simulink model "SSi_tracking_test_2024"  (R2024b)
settings: Solver=ode1  StartTime=0.0  StopTime=10  FixedStep=0.002  RelTol=1e-3  EnableMultiTasking=on
PostLoadFcn:
  | qc_set_target_type(getConfigSet(bdroot, 'QUARC Default Target Configuration'));
undefined symbols (not defined in the file): Aobs_d, Bobs_d, Cobs_d, Dobs_d, HIL, init_cond4, K5d, ud_neg, ud_pos, V_sat
libraries: quarc_library x4, simulink_extras x1
settings Model: SimulationMode=external  ExtModeTrigDuration=5000  Creator=pmartin  LastModifiedBy=Student
settings SolverCC: AlgebraicLoopSolver=TrustRegion  PositivePriorityOrder=on
settings DataIOCC: LimitDataPoints=on  SaveFormat=Array  SignalLoggingSaveFormat=ModelDataLogs  ReturnWorkspaceOutputs=off
settings OptimizationCC: ExpressionDepthLimit=2147483647  InitFltsAndDblsToZero=on
settings DebuggingCC: SaveWithParameterizedLinksMsg=none  UnderspecifiedInitializationDetection=Classic  MergeDetectMultiDrivingBlocksExec=none  SolverPrmCheckMsg=warning  MultiTaskDSMMsg=warning  MultiTaskCondExecSysMsg=none  FcnCallInpInsideContextMsg=warning  UnconnectedInputMsg=warning  UnconnectedOutputMsg=warning  UnconnectedLineMsg=warning  StateNameClashWarn=warning  SFUnexpectedBacktrackingDiag=warning  SFNoUnconditionalDefaultTransitionDiag=warning  SFExecutionAtInitializationDiag=none  ArithmeticOperatorsInVariantConditions=warning
settings ModelReferenceCC: PropagateSignalLabelsOutOfModel=off
settings SFSimCC: SimUseLocalCustomCode=off  CustomCodeUndefinedFunction=UseInterfaceOnly
settings RTWCC: Description=QUARC Win64 Target Using Toolchain  SystemTargetFile=quarc_win64.tlc  TemplateMakefile=quarc_default_tmf  RTWUseLocalCustomCode=off  Toolchain=QUARC win64 | nmake (64-bit Windows)  BuildConfiguration=Faster Runs  GPUComputeCapability=3.5
settings CodeAppCC: StateflowObjectComments=on
settings STFCustomTargetCC: ModelReferenceCompliant=off  CombineOutputUpdateFcns=on  MatFileLogging=on  UseToolchainInfoCompliant=on  SystemTargetFile=quarc_win64.tlc
settings GRTTargetCC: TargetLangStandard=C89/C90 (ANSI)  ModelReferenceCompliant=off  ParMdlRefBuildCompliant=off  CompOptLevelCompliant=off  ConcurrentExecutionCompliant=off  CPPClassGenCompliant=off  ExtMode=on  ExtModeMexFile=quarc_comm  ExtModeMexArgs='-w -uri %u'
settings ConfigComp: CovMetricSettings=dw  CovSaveCumulativeToWorkspaceVar=on  CovSaveSingleToWorkspaceVar=on  CovExternalEMLEnable=off

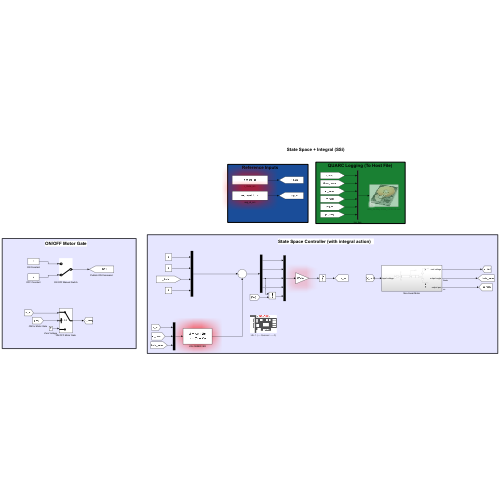
[thumbnail: Simulink's stored preview of the top-level diagram]
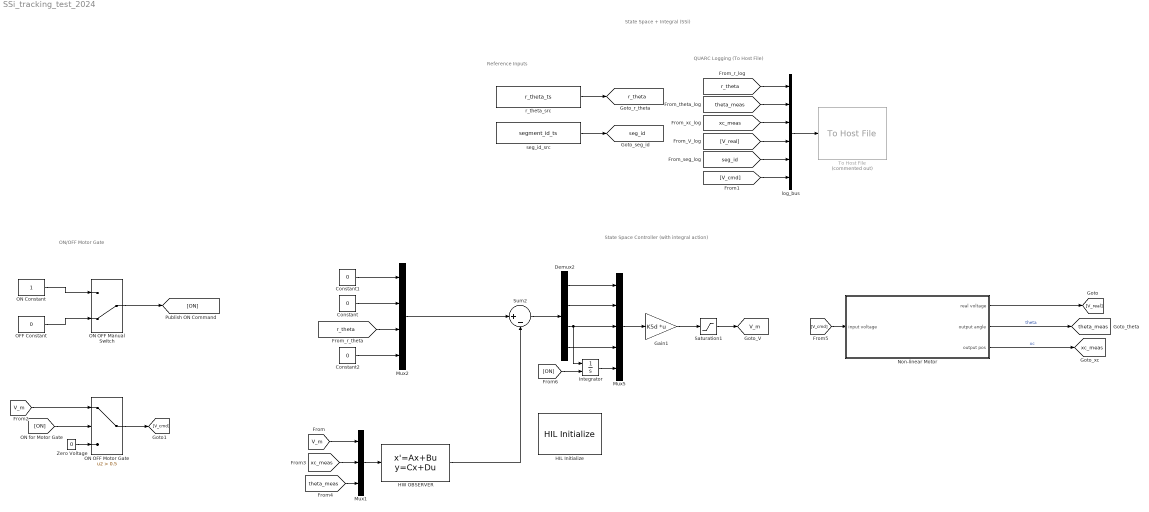
== system SSi_tracking_test_2024 ==
  note: State Space Controller (with integral action)
  note: State Space + Integral (SSi)
  note: Reference Inputs
  note: QUARC Logging (To Host File)
  note: ON/OFF Motor Gate
  Constant : Constant  Value=0
  Constant1 : Constant  Value=0
  Constant2 : Constant  Value=0
  Demux2 : Demux
  Gain1 : Gain  Gain=K5d  Multiplication=Matrix(K*u)
  HIL Initialize : quarc_library/Data Acquisition/Generic/Configuration/HIL Initialize  object_name=HIL-1  board_type=---- Quanser ----  board_number=0  board_options=d0=digital;d1=digital;led=auto;update_rate=normal  exclusive=off  active=off  hardware_clocks=[0:2]  clock_modes=[]  initial_clock_frequencies=[]  set_clock_params_at_start=off  set_clock_params_at_switch_in=off  set_clock_frequencies_at_start=off  set_clock_frequencies_at_switch_in=off  analog_input_channels=[0:1]  analog_input_configurations=[]  analog_input_maximums=10  analog_input_minimums=-10  set_analog_input_params_at_start=on  set_analog_input_params_at_switch_in=off  analog_output_channels=[0:1]  analog_output_maximums=10  analog_output_minimums=-10  initial_analog_outputs=[0]  final_analog_outputs=[0]  watchdog_analog_outputs=0  set_analog_output_params_at_start=on  set_analog_output_params_at_switch_in=off  set_analog_outputs_at_start=on  set_analog_outputs_at_switch_in=off  set_analog_outputs_at_terminate=on  set_analog_outputs_at_switch_out=off  set_analog_outputs_on_watchdog=off  digital_input_channels=[]  digital_output_channels=[0:7]  digital_output_configuration=[]  initial_digital_outputs=[0]  final_digital_outputs=[0]  watchdog_digital_outputs=[0]  set_digital_output_params_at_start=off  set_digital_output_params_at_switch_in=off  set_digital_outputs_at_start=on  set_digital_outputs_at_switch_in=off  set_digital_outputs_at_terminate=on  set_digital_outputs_at_switch_out=off  set_digital_outputs_on_watchdog=off  encoder_channels=[0:1]  quadrature=[4]  encoder_filter_frequency=[]  initial_encoder_counts=[0]  set_encoder_params_at_start=on  set_encoder_params_at_switch_in=off  set_encoder_counts_at_start=on  set_encoder_counts_at_switch_in=off  pwm_channels=[]  pwm_modes=[0]  pwm_frequency=1/0.020  pwm_configuration=[]  pwm_alignment=[]  pwm_polarity=[]  pwm_leading_deadband=[]  pwm_trailing_deadband=[]  initial_pwm_outputs=[0]  final_pwm_outputs=[0]  watchdog_pwm_outputs=[0]  set_pwm_params_at_start=on  set_pwm_params_at_switch_in=off  set_pwm_outputs_at_start=on  set_pwm_outputs_at_switch_in=off  set_pwm_outputs_at_terminate=on  set_pwm_outputs_at_switch_out=off  set_pwm_outputs_on_watchdog=off  other_output_channels=[]  initial_other_outputs=[]  final_other_outputs=[]  watchdog_other_outputs=[]  set_other_outputs_at_start=off  set_other_outputs_at_switch_in=off  set_other_outputs_at_terminate=off  set_other_outputs_at_switch_out=off  set_other_outputs_on_watchdog=off
  HW OBSERVER : StateSpace  A=Aobs_d  B=Bobs_d  C=Cobs_d  D=Dobs_d  InitialCondition=init_cond4
  Integrator : Integrator  ExternalReset=rising
  Mux1 : Mux  Inputs=3
  Mux2 : Mux
  Mux5 : Mux  Inputs=5
  Non-linear Motor : Subsystem
  OFF Constant : Constant  Value=0
  ON Constant : Constant
  ON OFF Manual Switch : ManualSwitch  CurrentSetting=0
  ON OFF Motor Gate : Switch  Criteria=u2 > Threshold  Threshold=0.5  SaturateOnIntegerOverflow=off  InputSameDT=off
  Saturation1 : Saturate  UpperLimit=6  LowerLimit=-6
  Sum2 : Sum  Inputs=|+-
  To Host File : quarc_library/Sinks/To Host/To Host File  Commented=on  source=Specify via dialog (do not evaluate)  file_name=data_%{date}_%{time}.mat  variable_name=data  decimation=1  sample_time=-1  file_format=MAT-file v.4  options=No header or footer  append=off  final_file_name=data_26-May-2026_14-35-08.mat  encoding=Default  bitrate=0
  Zero Voltage : Constant  Value=0
  log_bus : Mux  Inputs=6
  r_theta_src : FromWorkspace  VariableName=r_theta_ts  OutputAfterFinalValue=Holding final value
  seg_id_src : FromWorkspace  VariableName=segment_id_ts  Interpolate=off  OutputAfterFinalValue=Holding final value
  tag scope: V_m=global, r_theta=global, seg_id=global, theta_meas=global, xc_meas=global
  wires:
  Mux2/1 -> Sum2/1
  Constant1/1 -> Mux2/1
  Constant/1 -> Mux2/2
  Constant2/1 -> Mux2/4
  Saturation1/1 -> [V_m]
  HW OBSERVER/1 -> Sum2/2
  Mux1/1 -> HW OBSERVER/1
  Mux5/1 -> Gain1/1
  Demux2/4 -> Mux5/4
  Demux2/3 -> Integrator/1, Mux5/3
  Demux2/2 -> Mux5/2
  Demux2/1 -> Mux5/1
  Sum2/1 -> Demux2/1
  r_theta_src/1 -> [r_theta]
  seg_id_src/1 -> [seg_id]
  [r_theta] -> Mux2/3
  [r_theta] -> log_bus/1
  [theta_meas] -> log_bus/2
  [xc_meas] -> log_bus/3
  [V_real] -> log_bus/4
  [seg_id] -> log_bus/5
  log_bus/1 -> To Host File/1
  Gain1/1 -> Saturation1/1
  [V_m] -> Mux1/1
  Non-linear Motor/1(real voltage) -> [V_real]
  [V_cmd] -> log_bus/6
  Non-linear Motor/2(output angle) -> [theta_meas]  "theta"
  Non-linear Motor/3(output pos) -> [xc_meas]  "xc"
  [xc_meas] -> Mux1/2
  [theta_meas] -> Mux1/3
  Integrator/1 -> Mux5/5
  ON OFF Manual Switch/1 -> [ON]
  ON OFF Motor Gate/1 -> [V_cmd]
  ON Constant/1 -> ON OFF Manual Switch/1
  Zero Voltage/1 -> ON OFF Motor Gate/3
  [V_m] -> ON OFF Motor Gate/1
  OFF Constant/1 -> ON OFF Manual Switch/2
  [ON] -> ON OFF Motor Gate/2
  [V_cmd] -> Non-linear Motor/1(input voltage)
  [ON] -> Integrator/2

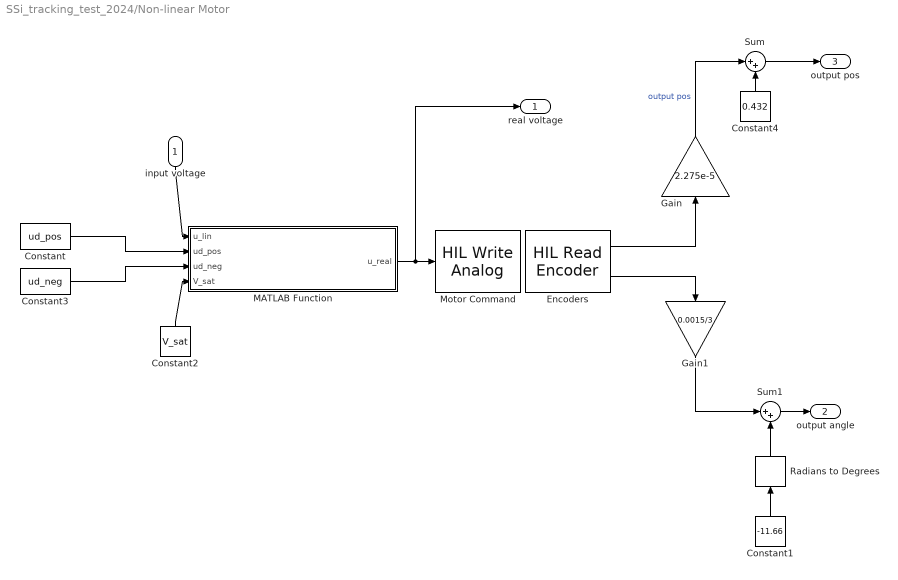
== system SSi_tracking_test_2024/Non-linear Motor ==
  input voltage : Inport
  Constant : Constant  Value=ud_pos
  Constant1 : Constant  Value=-11.66
  Constant2 : Constant  Value=V_sat
  Constant3 : Constant  Value=ud_neg
  Constant4 : Constant  Value=0.432
  Encoders : quarc_library/Data Acquisition/Generic/Immediate I//O/HIL Read Encoder  object_name=HIL-1  channels=[0,1]  sample_time=qc_get_step_size  active=on  vector_output=off  data_type_mode=Inherit via back propagation  data_type=double
  Gain : Gain  Gain=2.275e-5
  Gain1 : Gain  Gain=0.0015/3
  MATLAB Function : MATLAB Function  TreatAsAtomicUnit=on
  Motor Command : quarc_library/Data Acquisition/Generic/Immediate I//O/HIL Write Analog  object_name=HIL-1  channels=0  sample_time=-1  active=off  vector_input=off
  Radians to Degrees : simulink_extras/Transformations/Radians to Degrees
  Sum : Sum  Inputs=|++
  Sum1 : Sum  Inputs=|++
  real voltage : Outport
  output angle : Outport  Port=2
  output pos : Outport  Port=3
  wires:
  Encoders/1 -> Gain/1
  input voltage/1 -> MATLAB Function/1(u_lin)
  MATLAB Function/1(u_real) -> real voltage/1, Motor Command/1
  Constant/1 -> MATLAB Function/2(ud_pos)
  Constant3/1 -> MATLAB Function/3(ud_neg)
  Constant2/1 -> MATLAB Function/4(V_sat)
  Encoders/2 -> Gain1/1
  Gain/1 -> Sum/1  "output pos"
  Sum/1 -> output pos/1
  Gain1/1 -> Sum1/1
  Sum1/1 -> output angle/1
  Constant1/1 -> Radians to Degrees/1
  Radians to Degrees/1 -> Sum1/2
  Constant4/1 -> Sum/2

== matlab function SSi_tracking_test_2024/Non-linear Motor/MATLAB Function ==
  data: u_lin input; u_real output; ud_pos input; ud_neg input; V_sat input
function u_real = non_linear_deadzone(u_lin, ud_pos, ud_neg, V_sat)

epsilon = 0.1;

if u_lin > epsilon
    u_real = u_lin + ud_pos;
    
elseif u_lin < -epsilon
    u_real = u_lin - ud_neg;
    
else
    u_real = 0;
end

if u_real > V_sat
    u_real = V_sat;
elseif u_real < -V_sat
    u_real = -V_sat;
end
